simulink library "atc"  (Simulink 8.1)
settings: Solver=ode45  StartTime=0.0  StopTime=10.0  RelTol=1e-3
undefined symbols (not defined in the file or in its folder): KJUD_AEBConsideredDecel_mps2, KJUD_DecelThreshBraking_mps2
libraries: pbnbs x1, pbbs_new x1
settings Model: Creator=xsellart  LastModifiedBy=tescamilla

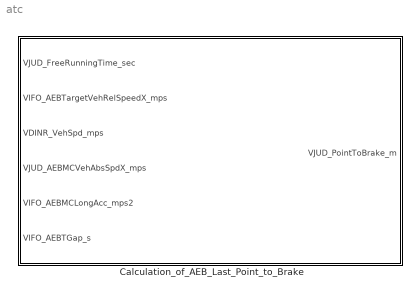
== system atc ==
  Calculation_of_AEB_Last_Point_to_Brake : Subsystem

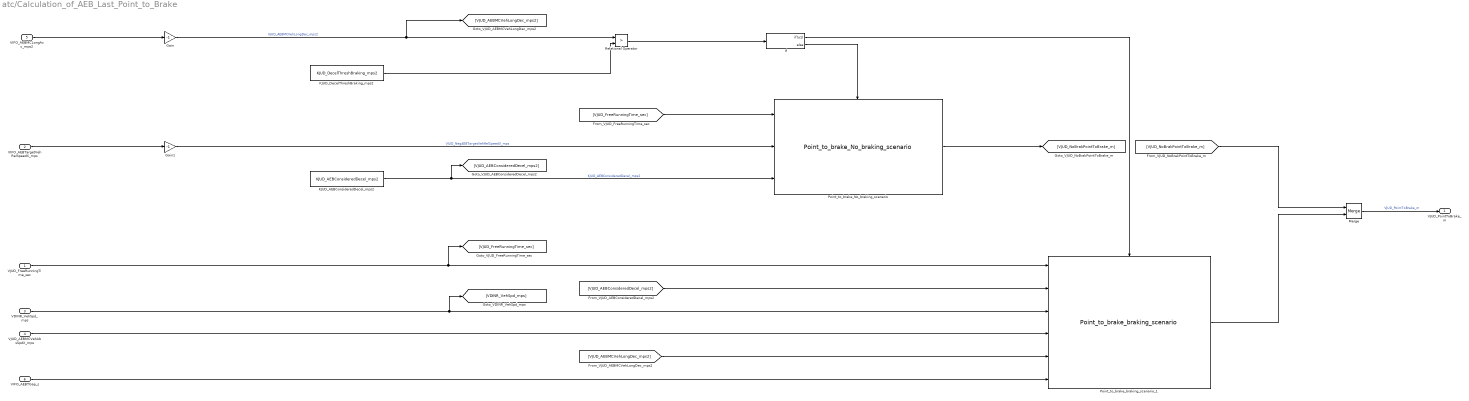
== system atc/Calculation_of_AEB_Last_Point_to_Brake ==
  VJUD_FreeRunningTime_sec : Inport
  VIFO_AEBTargetVehRelSpeedX_mps : Inport  Port=2
  VDINR_VehSpd_mps : Inport  Port=3
  VJUD_AEBMCVehAbsSpdX_mps : Inport  Port=4
  VIFO_AEBMCLongAcc_mps2 : Inport  Port=5
  VIFO_AEBTGap_s : Inport  Port=6
  Gain : Gain  Gain=-1  OutDataTypeStr=single
  Gain1 : Gain  Gain=-1  OutDataTypeStr=single
  If : If  IfExpression=u1
  KJUD_AEBConsideredDecel_mps2 : Constant  Value=KJUD_AEBConsideredDecel_mps2
  KJUD_DecelThreshBraking_mps2 : Constant  Value=KJUD_DecelThreshBraking_mps2  OutDataTypeStr=single
  Merge : Merge
  Point_to_brake_No_braking_scenario : pbnbs/Point_to_brake_No_braking_scenario
  Point_to_brake_braking_scenario_1 : pbbs_new/Point_to_brake_braking_scenario
  Relational Operator : RelationalOperator  Operator=>  OutDataTypeStr=boolean
  VJUD_PointToBrake_m : Outport
  wires:
  KJUD_DecelThreshBraking_mps2/1 -> Relational Operator/2
  VIFO_AEBTargetVehRelSpeedX_mps/1 -> Gain1/1
  Gain/1 -> [VJUD_AEBMCVehLongDec_mps2], Relational Operator/1  "VJUD_AEBMCVehLongDec_mps2"
  Relational Operator/1 -> If/1
  [VJUD_AEBConsideredDecel_mps2] -> Point_to_brake_braking_scenario_1/2
  VJUD_FreeRunningTime_sec/1 -> [VJUD_FreeRunningTime_sec], Point_to_brake_braking_scenario_1/1
  If/1 -> Point_to_brake_braking_scenario_1/Action
  [VJUD_AEBMCVehLongDec_mps2] -> Point_to_brake_braking_scenario_1/5
  [VJUD_FreeRunningTime_sec] -> Point_to_brake_No_braking_scenario/1
  Gain1/1 -> Point_to_brake_No_braking_scenario/2  "VJUD_NegAEBTargetVehRelSpeedX_mps"
  KJUD_AEBConsideredDecel_mps2/1 -> Point_to_brake_No_braking_scenario/3, [VJUD_AEBConsideredDecel_mps2]  "KJUD_AEBConsideredDecel_mps2"
  If/2 -> Point_to_brake_No_braking_scenario/Action
  Point_to_brake_No_braking_scenario/1 -> [VJUD_NoBrakPointToBrake_m]
  [VJUD_NoBrakPointToBrake_m] -> Merge/1
  Point_to_brake_braking_scenario_1/1 -> Merge/2
  Merge/1 -> VJUD_PointToBrake_m/1  "VJUD_PointToBrake_m"
  VIFO_AEBMCLongAcc_mps2/1 -> Gain/1
  VJUD_AEBMCVehAbsSpdX_mps/1 -> Point_to_brake_braking_scenario_1/4
  VDINR_VehSpd_mps/1 -> Point_to_brake_braking_scenario_1/3, [VDINR_VehSpd_mps]
  VIFO_AEBTGap_s/1 -> Point_to_brake_braking_scenario_1/6
